simulink model "Dyn_6DoF_v2_0_R2015B"  (R2015b)
settings: Solver=ode4  SolverMode=SingleTasking  StartTime=0.0  StopTime=simInit.TSIM  FixedStep=simInit.dt  MaxStep=simInit.dt  RelTol=1e-3
InitFcn:
  | close all
undefined symbols (not defined in the file): act, base_windspeed, constr, DE2019, DiscIntNeverNeededParam, ENVMT, Lbooth, loiterStates, omega_rate_max, params, simInit, T, winchParameter
libraries: simulink x41, simulink_extras x4, dspsigops x1
(part 1 of 6)
Description:
  | % Copyright 2020 Delft University of Technology
  | %
  | % Licensed under the Apache License, Version 2.0 (the "License");
  | % you may not use this file except in compliance with the License.
  | % You may obtain a copy of the License at
  | %
  | %      http://www.apache.org/licenses/LICENSE-2.0
  | %
  | % Unless required by applicable law or agreed to in writing, software
  | % distributed under the License is distributed on an "AS IS" BASIS,
  | % WITHOUT WARRANTIES OR CONDITIONS OF ANY KIND, either express or implied.
  | % See the License for the specific language governing permissions and
  | % limitations under the License.
settings Model: SimulationMode=accelerator  NumberOfSteps=50  ExtModeTrigDuration=100  Creator=Sebastian  LastModifiedBy=dylaneijkelhof
settings SolverCC: SolverJacobianMethodControl=FullAnalytical
settings DataIOCC: InitialState=testPoint  LimitDataPoints=off  SaveFormat=Structure  SignalLogging=off  DSMLogging=off  SaveTime=off  StateSaveName=tmp_raccel_xout  SignalLoggingName=logged_signals
settings OptimizationCC: BlockReduction=off  EfficientMapNaN2IntZero=off
settings DebuggingCC: ArtificialAlgebraicLoopMsg=none  SaveWithDisabledLinksMsg=none  SaveWithParameterizedLinksMsg=none  MaskedZcDiagnostic=none  IgnoredZcDiagnostic=none  InheritedTsInSrcMsg=none  TasksWithSamePriorityMsg=none  SigSpecEnsureSampleTimeMsg=none  ParameterPrecisionLossMsg=none  UnconnectedInputMsg=none  UnconnectedOutputMsg=none  UnconnectedLineMsg=none  BusObjectLabelMismatch=none  RootOutportRequireBusObject=none  AllowSymbolicDim=on  UnknownTsInhSupMsg=none  ModelReferenceDataLoggingMessage=none  ModelReferenceSymbolNameMessage=none  InitInArrayFormatMsg=none  SFUnusedDataAndEventsDiag=none  SFUnexpectedBacktrackingDiag=none  SFInvalidInputDataAccessInChartInitDiag=none  SFNoUnconditionalDefaultTransitionDiag=none  SFTransitionOutsideNaturalParentDiag=none  SFUnconditionalTransitionShadowingDiag=none  SFUndirectedBroadcastEventsDiag=none  SFTransitionActionBeforeConditionDiag=none
settings HardwareCC: ProdBitPerLong=64  ProdLongLongMode=on  ProdHWDeviceType=Custom Processor->Custom Processor  TargetBitPerLong=64  TargetBitPerPointer=64  TargetLargestAtomicFloat=Float  TargetLongLongMode=on  TargetIntDivRoundTo=Zero  TargetEndianess=LittleEndian  TargetWordSize=64  TargetHWDeviceType=Custom Processor->MATLAB Host Computer
settings RTWCC: RTWUseLocalCustomCode=on
settings CodeAppCC: MaxIdLength=128
settings GRTTargetCC: CombineOutputUpdateFcns=off  GRTInterface=on
settings ConfigComp: CovModelRefEnable=Off
settings SimscapeCC: SimscapeNormalizeSystem=off

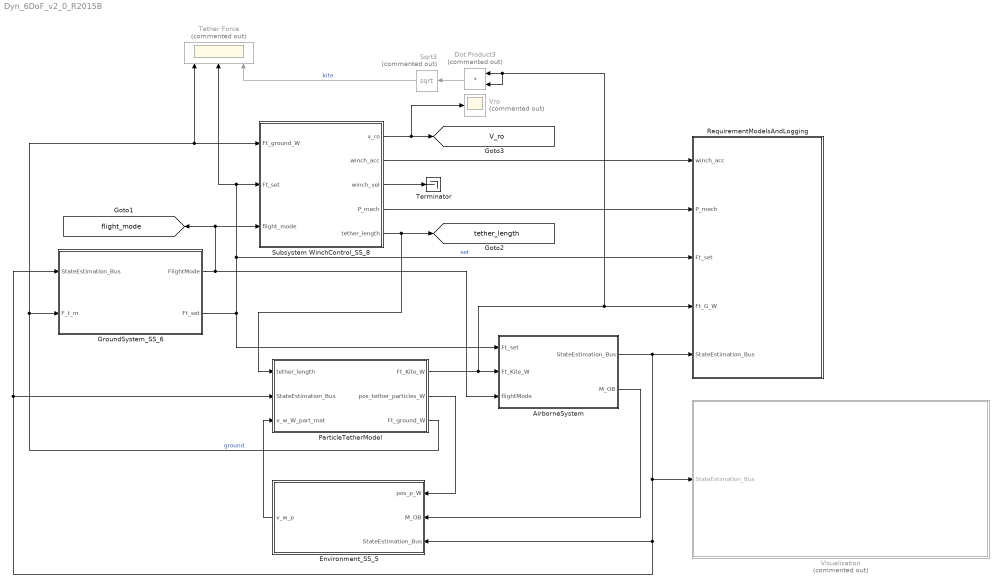
== system Dyn_6DoF_v2_0_R2015B ==
  AirborneSystem : Subsystem
  Dot Product3 : DotProduct  Commented=on  InputSameDT=on  OutDataTypeStr=Inherit: Inherit via internal rule
  Environment_SS_5 : Subsystem
  GroundSystem_SS_6 : Subsystem
  ParticleTetherModel : Subsystem
  RequirementModelsAndLogging : Subsystem  mask{log_sample_time=0.2}
  Sqrt3 : Sqrt  Commented=on  SaturateOnIntegerOverflow=on
  Subsystem WinchControl_SS_8 : Subsystem
  Terminator : Terminator
  Tether Force : Scope  Commented=on  NumInputPorts=3
  Visualisation : Subsystem  Commented=on  mask{sample_time_vis=1}
      mask prompts: sample_time_vis "sampletime"
      mask Display: image('DE2019_Aircraft.jpeg')
  Vro : Scope  Commented=on
  tag scope: V_ro=global, flight_mode=global, tether_length=global
  wires:
  GroundSystem_SS_6/1(FlightMode) -> AirborneSystem/3(flightMode), Subsystem WinchControl_SS_8/3(flight_mode), [flight_mode]
  GroundSystem_SS_6/2(Ft_set) -> Subsystem WinchControl_SS_8/2(Ft_set), Tether Force/2, RequirementModelsAndLogging/3(Ft_set), AirborneSystem/1(Ft_set)  "set"
  AirborneSystem/2(M_OB) -> Environment_SS_5/2(M_OB)
  AirborneSystem/1(StateEstimation_Bus) -> RequirementModelsAndLogging/5(StateEstimation_Bus), Environment_SS_5/3(StateEstimation_Bus), GroundSystem_SS_6/1(StateEstimation_Bus), ParticleTetherModel/2(StateEstimation_Bus), Visualisation/1(StateEstimation_Bus)
  ParticleTetherModel/2(pos_tether_particles_W) -> Environment_SS_5/1(pos_p_W)
  Environment_SS_5/1(v_w_p) -> ParticleTetherModel/3(v_w_W_part_mat)
  Subsystem WinchControl_SS_8/1(v_ro) -> Vro/1, [V_ro]
  ParticleTetherModel/3(Ft_ground_W) -> GroundSystem_SS_6/2(F_t_m), Subsystem WinchControl_SS_8/1(Ft_ground_W), Tether Force/1  "ground"
  Subsystem WinchControl_SS_8/3(winch_vel) -> Terminator/1
  Subsystem WinchControl_SS_8/2(winch_acc) -> RequirementModelsAndLogging/1(winch_acc)
  Subsystem WinchControl_SS_8/4(P_mech) -> RequirementModelsAndLogging/2(P_mech)
  Subsystem WinchControl_SS_8/5(tether_length) -> [tether_length], ParticleTetherModel/1(tether_length)
  Sqrt3/1 -> Tether Force/3  "kite"
  Dot Product3/1 -> Sqrt3/1
  ParticleTetherModel/1(Ft_Kite_W) -> RequirementModelsAndLogging/4(Ft_G_W), Dot Product3/2, Dot Product3/1, AirborneSystem/2(Ft_Kite_W)

== system Dyn_6DoF_v2_0_R2015B/AirborneSystem ==
  Ft_set : Inport
  Ft_Kite_W : Inport  Port=2
  flightMode : Inport  Port=3
  6DoFDynamics : Subsystem
  Dot Product : DotProduct  InputSameDT=on  OutDataTypeStr=Inherit: Inherit via internal rule
  FlightControlSystem : Subsystem
  ForcesAndTorques : Subsystem
  Sqrt : Sqrt  SaturateOnIntegerOverflow=on
  StateEstimation_Bus : Outport
  M_OB : Outport  Port=2
  wires:
  6DoFDynamics/2(StateEstimation_Bus) -> FlightControlSystem/4(StateEstimation_Bus), ForcesAndTorques/3(StateEstimation_Bus), StateEstimation_Bus/1  "StateEstimation_Bus"
  6DoFDynamics/1(M_OB) -> M_OB/1
  Ft_Kite_W/1 -> 6DoFDynamics/1(F_t_W), Dot Product/2, Dot Product/1
  Dot Product/1 -> Sqrt/1
  Ft_set/1 -> FlightControlSystem/2(Ft_set)
  Sqrt/1 -> FlightControlSystem/3(Ft_tot_kite)
  ForcesAndTorques/1(F_a_B) -> 6DoFDynamics/2(F_a_B), FlightControlSystem/1(F_a_B)
  FlightControlSystem/2(throttle/brake) -> ForcesAndTorques/2(throttle/brake)
  ForcesAndTorques/2(F_p_B) -> 6DoFDynamics/3(F_p_B)
  ForcesAndTorques/3(M_a_B) -> 6DoFDynamics/4(Torques), FlightControlSystem/5(M_a_B)
  FlightControlSystem/1(u_controlsurfaces) -> ForcesAndTorques/1(u_cmd)
  flightMode/1 -> FlightControlSystem/6(fm)

== system Dyn_6DoF_v2_0_R2015B/Environment_SS_5 ==
  note: Tether
  note: Kite
  note: note: wind field calc occurs twice, here and in windshear
  pos_p_W : Inport
  M_OB : Inport  Port=2
  StateEstimation_Bus : Inport  Port=3
  Bus Selector : BusSelector  OutputSignals=pos_G_O_m
  Constant4 : Constant  Value=ENVMT.windDirection_rad
  Delay : Delay  DelayLength=1  InitialCondition=zeros(3,1)
  Gain : Gain  Gain=-1
  Gain1 : Gain  Gain=-1
  MATLAB Function : MATLAB Function  TreatAsAtomicUnit=on
  MATLAB Function1 : MATLAB Function  TreatAsAtomicUnit=on
  Product : Product  Multiplication=Matrix(*)
  Reshape1 : Reshape  OutputDimensionality=Column vector (2-D)
  Selector : Selector  InputPortWidth=3  IndexOptions=Index vector (dialog)  Indices=3  OutputSizes=1
  Wdeg2 : Constant  Value=base_windspeed  OutDataTypeStr=Inherit: Inherit via back propagation
  Windshear : Subsystem
  wind_field_calc : Subsystem
  v_w_p : Outport
  tag scope: vel_W_W=global
  wires:
  wind_field_calc/1(Windspeed_altitude) -> MATLAB Function1/1(v_w_u)
  Wdeg2/1 -> wind_field_calc/2(Base_windspeed)
  Delay/1 -> [vel_W_W]
  MATLAB Function1/1(v_w_p_mat) -> v_w_p/1
  pos_p_W/1 -> wind_field_calc/1(Altitude)
  Reshape1/1 -> Delay/1
  Constant4/1 -> MATLAB Function/2(wind_direction_rad)
  Gain/1 -> Windshear/2(altitude)
  Gain1/1 -> Product/2
  Windshear/1(V_shear_mDs) -> Gain1/1
  M_OB/1 -> Windshear/1(DCM), Product/1
  Product/1 -> MATLAB Function/1(vec_O)
  StateEstimation_Bus/1 -> Bus Selector/1
  MATLAB Function/1(vec_W) -> Reshape1/1
  Selector/1 -> Gain/1
  Bus Selector/1 -> Selector/1  "<pos_G_O_m>"

== system Dyn_6DoF_v2_0_R2015B/GroundSystem_SS_6 ==
  StateEstimation_Bus : Inport
  F_t_m : Inport  Port=2
  Bus Selector : BusSelector  OutputSignals=pos_G_W,airdata,longlat,pathangles_k
  Demux : Demux  Outputs=2
  Demux1 : Demux  Outputs=2
  GroundControl : Subsystem
  Selector : Selector  InputPortWidth=3  IndexOptions=Index vector (dialog)  Indices=1  OutputSizes=1
  Selector1 : Selector  InputPortWidth=3  IndexOptions=Index vector (dialog)  Indices=1  OutputSizes=1
  Selector3 : Selector  InputPortWidth=2  IndexOptions=Index vector (dialog)  Indices=1  OutputSizes=1
  StateMachine : Subsystem
  Terminator : Terminator
  FlightMode : Outport
  Ft_set : Outport  Port=2
  tag scope: phi0_update=global
  wires:
  Demux1/1 -> StateMachine/9(Chi)
  Demux1/2 -> Terminator/1
  Bus Selector/4 -> Demux1/1  "<pathangles_k>"
  GroundControl/2(lat_init) -> StateMachine/8(lat_init)
  Selector3/1 -> GroundControl/2(long)
  GroundControl/1(path_update) -> Selector1/1, StateMachine/5(path_update)
  Selector1/1 -> [phi0_update]
  StateMachine/1(FlightMode) -> FlightMode/1, GroundControl/1(flightMode)
  Bus Selector/3 -> Selector3/1, Demux/1  "<longlat>"
  F_t_m/1 -> StateMachine/7(F_t_m)
  [cross_track_error] -> StateMachine/6(cross_track_error)
  Demux/2 -> StateMachine/4(lattitude)
  StateMachine/2(Ft_set) -> Ft_set/1
  Demux/1 -> StateMachine/3(longitude)
  StateEstimation_Bus/1 -> Bus Selector/1
  Bus Selector/1 -> StateMachine/1(pos_W)  "<pos_G_W>"
  Bus Selector/2 -> Selector/1  "<airdata>"
  Selector/1 -> StateMachine/2(Va)

== system Dyn_6DoF_v2_0_R2015B/ParticleTetherModel ==
  tether_length : Inport
  StateEstimation_Bus : Inport  Port=2
  v_w_W_part_mat : Inport  Port=3
  Bus Selector : BusSelector  OutputSignals=pos_G_W,vel_W
  Dot Product2 : DotProduct  Commented=on  InputSameDT=on  OutDataTypeStr=Inherit: Inherit via internal rule
  Selector : Selector  NumberOfDimensions=2  InputPortWidth=3  IndexOptions=Index vector (dialog),Select all  Indices=1,1  OutputSizes=1,1
  Selector4 : Selector  NumberOfDimensions=2  InputPortWidth=3  IndexOptions=Index vector (dialog),Select all  Indices=2,1  OutputSizes=1,1
  Selector5 : Selector  NumberOfDimensions=2  InputPortWidth=3  IndexOptions=Index vector (dialog),Select all  Indices=3,1  OutputSizes=1,1
  Sqrt2 : Sqrt  Commented=on  SaturateOnIntegerOverflow=on
  Tether_SS_7 : Subsystem
  Transpose : Math  Operator=transpose  SaturateOnIntegerOverflow=on
  Transpose1 : Math  Operator=transpose  SaturateOnIntegerOverflow=on
  Transpose2 : Math  Operator=transpose  SaturateOnIntegerOverflow=on
  error tether : Scope  Commented=on
  Ft_Kite_W : Outport
  pos_tether_particles_W : Outport  Port=2
  Ft_ground_W : Outport  Port=3
  tag scope: p_t_x=global, p_t_y=global, p_t_z=global
  wires:
  v_w_W_part_mat/1 -> Tether_SS_7/3(windVel)
  StateEstimation_Bus/1 -> Bus Selector/1
  Bus Selector/1 -> Tether_SS_7/1(pos_G_W)  "<pos_G_W>"
  Bus Selector/2 -> Tether_SS_7/2(vel_W)  "<vel_W>"
  Selector4/1 -> Transpose1/1
  Selector5/1 -> Transpose2/1
  Selector/1 -> Transpose/1
  Transpose/1 -> [p_t_x]
  Transpose1/1 -> [p_t_y]
  Transpose2/1 -> pos_tether_particles_W/1, [p_t_z]
  Tether_SS_7/4(Error_3D) -> Dot Product2/2, Dot Product2/1
  Tether_SS_7/1(x tether W) -> Selector/1, Selector5/1, Selector4/1
  Dot Product2/1 -> Sqrt2/1
  Sqrt2/1 -> error tether/1
  Tether_SS_7/2(Ft_Ground) -> Ft_ground_W/1
  Tether_SS_7/3(Ft_Kite) -> Ft_Kite_W/1
  tether_length/1 -> Tether_SS_7/4(tetherLength)

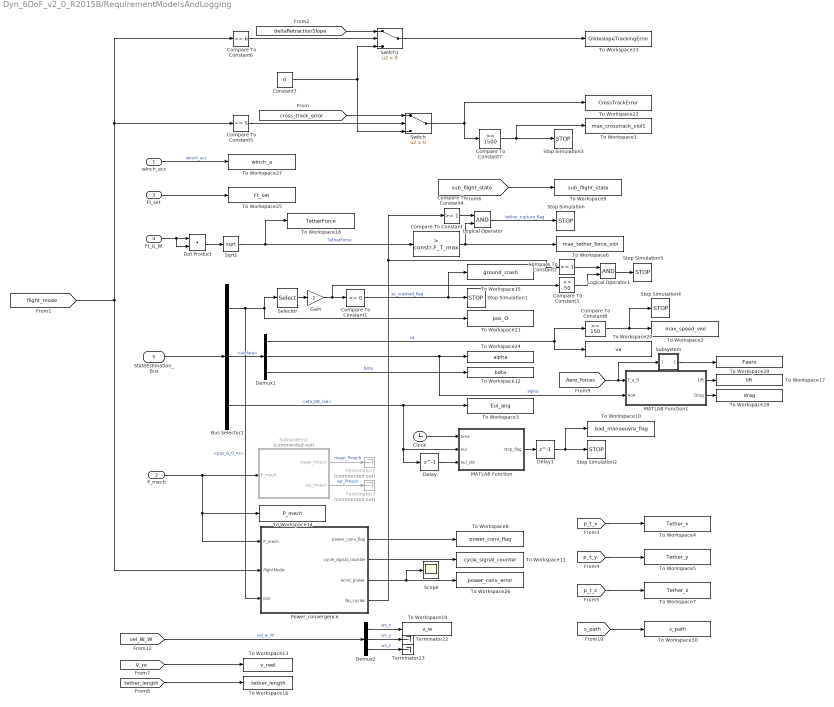
== system Dyn_6DoF_v2_0_R2015B/RequirementModelsAndLogging ==
  winch_acc : Inport
  P_mech : Inport  Port=2
  Ft_set : Inport  Port=3
  Ft_G_W : Inport  Port=4
  StateEstimation_Bus : Inport  Port=5
  Bus Selector1 : BusSelector  OutputSignals=pos_G_O_m,airdata,eta_OB_rad
  Clock : Clock
  Compare To Constant : simulink/Logic and Bit Operations/Compare To Constant  relop=>  const=constr.F_T_max  OutDataTypeStr=boolean
  Compare To Constant1 : simulink/Logic and Bit Operations/Compare To Constant  relop=<=  const=0  OutDataTypeStr=boolean
  Compare To Constant2 : simulink/Logic and Bit Operations/Compare To Constant  relop=>=  const=1  OutDataTypeStr=boolean
  Compare To Constant3 : simulink/Logic and Bit Operations/Compare To Constant  relop=<=  const=50  OutDataTypeStr=boolean
  Compare To Constant4 : simulink/Logic and Bit Operations/Compare To Constant  relop=>=  const=1  OutDataTypeStr=boolean
  Compare To Constant5 : simulink/Logic and Bit Operations/Compare To Constant  relop===  const=5  OutDataTypeStr=boolean
  Compare To Constant6 : simulink/Logic and Bit Operations/Compare To Constant  relop===  const=6  OutDataTypeStr=boolean
  Compare To Constant7 : simulink/Logic and Bit Operations/Compare To Constant  relop=>=  const=1500  OutDataTypeStr=boolean
  Compare To Constant8 : simulink/Logic and Bit Operations/Compare To Constant  relop=>=  const=150  OutDataTypeStr=boolean
  Constant7 : Constant  Value=0
  Delay : Delay  DelayLength=1  InitialCondition=zeros(3,1)
  Delay1 : Delay  DelayLength=1
  Demux1 : Demux  Outputs=3
  Demux2 : Demux  Outputs=3
  Dot Product : DotProduct  InputSameDT=on  OutDataTypeStr=Inherit: Inherit via internal rule
  Gain : Gain  Gain=-1
  Logical Operator : Logic  AllPortsSameDT=off  OutDataTypeStr=boolean
  Logical Operator1 : Logic  AllPortsSameDT=off  OutDataTypeStr=boolean
  MATLAB Function : MATLAB Function  TreatAsAtomicUnit=on
  MATLAB Function1 : MATLAB Function  TreatAsAtomicUnit=on
  Power_convergence : Subsystem  mask{sample_time=simInit.Ts_power_conv_check, threshold=130000, min_cycles=3, pos_threshold=400}
      mask prompts: threshold "start_threshold"; min_cycles "minimum_cycles"; pos_threshold "maximum position distance"
  Scope : Scope
  Selector : Selector  InputPortWidth=3  IndexOptions=Index vector (dialog)  Indices=3  OutputSizes=1
  Sqrt1 : Sqrt  SaturateOnIntegerOverflow=on
  Stop Simulation{,1..5} (6 alike) : Stop
  Subsystem : Subsystem
      mask Display: disp('norm()')
  Subsystem2 : Subsystem  Commented=on
  Switch : Switch  Criteria=u2 > Threshold
  Switch1 : Switch  Criteria=u2 > Threshold
  Terminator1 : Terminator  Commented=on
  Terminator22 : Terminator
  Terminator23 : Terminator
  Terminator7 : Terminator  Commented=on
  To Workspace1 : ToWorkspace  VariableName=max_crosstrack_viol1  SampleTime=-1
      settings: MaxDataPoints=1
  To Workspace10 : ToWorkspace  VariableName=bad_manoeuvre_flag  SampleTime=-1
      settings: MaxDataPoints=1
  To Workspace11 : ToWorkspace  VariableName=cycle_signal_counter  SaveFormat=Timeseries  SampleTime=-1
      settings: MaxDataPoints=1  Save2DSignal=2-D array (concatenate along first dimension)
  To Workspace12 : ToWorkspace  VariableName=beta  SaveFormat=Timeseries  SampleTime=simInit.AttLoggingTs
      settings: Save2DSignal=2-D array (concatenate along first dimension)
  To Workspace13 : ToWorkspace  VariableName=v_reel  SaveFormat=Timeseries  SampleTime=simInit.PLoggingTs
  To Workspace14 : ToWorkspace  VariableName=P_mech  SaveFormat=Timeseries  SampleTime=simInit.PLoggingTs
  To Workspace15 : ToWorkspace  VariableName=ground_crash  SampleTime=-1
      settings: MaxDataPoints=1
  To Workspace16 : ToWorkspace  VariableName=tether_length  SaveFormat=Timeseries  SampleTime=simInit.AttLoggingTs
  To Workspace17 : ToWorkspace  VariableName=lift  SaveFormat=Timeseries  SampleTime=simInit.AttLoggingTs
      settings: Save2DSignal=2-D array (concatenate along first dimension)
  To Workspace18 : ToWorkspace  VariableName=TetherForce  SaveFormat=Timeseries  SampleTime=simInit.FtLoggingTs
  To Workspace19 : ToWorkspace  VariableName=v_w  SaveFormat=Timeseries  SampleTime=simInit.PLoggingTs
  To Workspace2 : ToWorkspace  VariableName=max_speed_viol  SampleTime=-1
      settings: MaxDataPoints=1
  To Workspace20 : ToWorkspace  VariableName=va  SaveFormat=Timeseries  SampleTime=simInit.AttLoggingTs
      settings: Save2DSignal=2-D array (concatenate along first dimension)
  To Workspace21 : ToWorkspace  VariableName=pos_O  SaveFormat=Timeseries  SampleTime=simInit.PLoggingTs
      settings: Save2DSignal=2-D array (concatenate along first dimension)
  To Workspace22 : ToWorkspace  VariableName=CrossTrackError  SaveFormat=Timeseries  SampleTime=simInit.CteLoggingTs
      settings: Save2DSignal=2-D array (concatenate along first dimension)
  To Workspace23 : ToWorkspace  VariableName=GlideslopeTrackingError  SaveFormat=Timeseries  SampleTime=simInit.GSLoggingTs
      settings: Save2DSignal=2-D array (concatenate along first dimension)
  To Workspace24 : ToWorkspace  VariableName=alpha  SaveFormat=Timeseries  SampleTime=simInit.AttLoggingTs
      settings: Save2DSignal=2-D array (concatenate along first dimension)
  To Workspace25 : ToWorkspace  VariableName=Ft_set  SaveFormat=Timeseries  SampleTime=simInit.FtLoggingTs
  To Workspace26 : ToWorkspace  VariableName=power_conv_error  SaveFormat=Timeseries  SampleTime=-1
      settings: Save2DSignal=2-D array (concatenate along first dimension)
  To Workspace27 : ToWorkspace  VariableName=winch_a  SaveFormat=Timeseries  SampleTime=simInit.PLoggingTs
  To Workspace28 : ToWorkspace  VariableName=drag  SaveFormat=Timeseries  SampleTime=simInit.AttLoggingTs
      settings: Save2DSignal=2-D array (concatenate along first dimension)
  To Workspace29 : ToWorkspace  VariableName=Faero  SaveFormat=Timeseries  SampleTime=simInit.AttLoggingTs
      settings: Save2DSignal=2-D array (concatenate along first dimension)
  To Workspace3 : ToWorkspace  VariableName=Eul_ang  SaveFormat=Timeseries  SampleTime=simInit.PLoggingTs
      settings: Save2DSignal=2-D array (concatenate along first dimension)
  To Workspace30 : ToWorkspace  VariableName=s_path  SaveFormat=Timeseries  SampleTime=simInit.PLoggingTs
      settings: Save2DSignal=2-D array (concatenate along first dimension)
  To Workspace4 : ToWorkspace  VariableName=Tether_x  SaveFormat=Timeseries  SampleTime=simInit.PLoggingTs
      settings: Save2DSignal=2-D array (concatenate along first dimension)
  To Workspace5 : ToWorkspace  VariableName=Tether_y  SaveFormat=Timeseries  SampleTime=simInit.PLoggingTs
      settings: Save2DSignal=2-D array (concatenate along first dimension)
  To Workspace6 : ToWorkspace  VariableName=max_tether_force_viol  SampleTime=-1
      settings: MaxDataPoints=1
  To Workspace7 : ToWorkspace  VariableName=Tether_z  SaveFormat=Timeseries  SampleTime=simInit.PLoggingTs
      settings: Save2DSignal=2-D array (concatenate along first dimension)
  To Workspace8 : ToWorkspace  VariableName=power_conv_flag  SampleTime=-1
      settings: MaxDataPoints=1
  To Workspace9 : ToWorkspace  VariableName=sub_flight_state  SaveFormat=Timeseries  SampleTime=simInit.FtLoggingTs
  wires:
  Bus Selector1/1 -> Power_convergence/3(pos), Selector/1, To Workspace21/1  "<pos_G_O_m>"
  Gain/1 -> Compare To Constant3/1, Compare To Constant1/1
  Compare To Constant1/1 -> To Workspace15/1, Stop Simulation1/1  "ac_crashed_flag"
  Selector/1 -> Gain/1
  winch_acc/1 -> To Workspace27/1  "winch_acc"
  Logical Operator/1 -> Stop Simulation/1  "tether_rupture_flag"
  Sqrt1/1 -> To Workspace18/1, Compare To Constant/1  "TetherForce"
  StateEstimation_Bus/1 -> Bus Selector1/1
  Power_convergence/1(power_conv_flag) -> To Workspace8/1
  Power_convergence/2(cycle_signal_counter) -> To Workspace11/1
  [vel_W_W] -> Demux2/1  "vel_w_W"
  Bus Selector1/2 -> Demux1/1  "<airdata>"
  Switch/1 -> To Workspace22/1, Compare To Constant7/1
  Subsystem2/1(mean_Pmech) -> Terminator1/1  "mean_Pmech"
  Subsystem2/2(var_Pmech) -> Terminator7/1  "var_Pmech"
  Demux1/1 -> To Workspace20/1, Compare To Constant8/1  "va"
  Demux1/2 -> MATLAB Function1/2(AoA), To Workspace24/1  "alpha"
  Demux1/3 -> To Workspace12/1  "beta"
  Demux2/3 -> Terminator23/1  "ws_z"
  Demux2/2 -> Terminator22/1  "ws_y"
  Demux2/1 -> To Workspace19/1  "ws_x"
  Ft_G_W/1 -> Dot Product/2, Dot Product/1
  Dot Product/1 -> Sqrt1/1
  Clock/1 -> MATLAB Function/1(time)
  Compare To Constant4/1 -> Logical Operator/1
  Compare To Constant/1 -> Logical Operator/2, To Workspace6/1
  [flight_mode] -> Compare To Constant6/1, Compare To Constant5/1, Power_convergence/2(flightMode)
  P_mech/1 -> Power_convergence/1(P_mech), To Workspace14/1, Subsystem2/1(P_mech)
  Compare To Constant5/1 -> Switch/2
  [cross_track_error] -> Switch/1
  Switch1/1 -> To Workspace23/1
  [deltaRetractionSlope] -> Switch1/1
  Compare To Constant6/1 -> Switch1/2
  Constant7/1 -> Switch1/3, Switch/3
  Ft_set/1 -> To Workspace25/1
  Power_convergence/3(error_power) -> Scope/1, To Workspace26/1
  Compare To Constant7/1 -> Stop Simulation3/1, To Workspace1/1
  Compare To Constant8/1 -> To Workspace2/1, Stop Simulation4/1
  Bus Selector1/3 -> Delay/1, MATLAB Function/2(eul), To Workspace3/1  "<eta_OB_rad>"
  [p_t_y] -> To Workspace5/1
  [p_t_x] -> To Workspace4/1
  [p_t_z] -> To Workspace7/1
  [sub_flight_state] -> To Workspace9/1
  Delay/1 -> MATLAB Function/3(eul_old)
  MATLAB Function/1(stop_flag) -> Delay1/1
  Delay1/1 -> Stop Simulation2/1, To Workspace10/1
  [V_ro] -> To Workspace13/1
  [tether_length] -> To Workspace16/1
  [Aero_forces] -> Subsystem/1(In1), MATLAB Function1/1(F_a_B)
  MATLAB Function1/1(Lift) -> To Workspace17/1
  MATLAB Function1/2(Drag) -> To Workspace28/1
  Power_convergence/4(No_cycles) -> Compare To Constant2/1, Compare To Constant4/1
  Compare To Constant2/1 -> Logical Operator1/1
  Compare To Constant3/1 -> Logical Operator1/2
  Logical Operator1/1 -> Stop Simulation5/1
  Subsystem/1(Out1) -> To Workspace29/1
  [s_path] -> To Workspace30/1

== system Dyn_6DoF_v2_0_R2015B/Subsystem WinchControl_SS_8 ==
  Ft_ground_W : Inport  OutDataTypeStr=double  PortDimensions=1
  Ft_set : Inport  Port=2  OutDataTypeStr=double  PortDimensions=1
  flight_mode : Inport  Port=3  OutDataTypeStr=double  PortDimensions=1
  Compare To Constant1 : simulink/Logic and Bit Operations/Compare To Constant  relop===  const=6  OutDataTypeStr=boolean
  Gain1 : Gain  Gain=winchParameter.radius
  Power : Scope
  Product : Product
  PureTorqueControl : Subsystem
  Reel-out speed : Scope
  Scope : Scope  Commented=on
  Winch acc : Scope
  WinchDynamics : Subsystem
  tether length : Scope
  v_ro : Outport  OutDataTypeStr=double  PortDimensions=1
  winch_acc : Outport  Port=2  OutDataTypeStr=double  PortDimensions=1
  winch_vel : Outport  Port=3  OutDataTypeStr=double  PortDimensions=1
  P_mech : Outport  Port=4  OutDataTypeStr=double  PortDimensions=1
  tether_length : Outport  Port=5  OutDataTypeStr=double  PortDimensions=1
  wires:
  Gain1/1 -> Product/2, Reel-out speed/1, v_ro/1
  WinchDynamics/2(theta_dot) -> PureTorqueControl/4(theta_dot), Gain1/1
  Ft_ground_W/1 -> PureTorqueControl/1(F_t_m_grnd), Product/1, WinchDynamics/1(for_tether_tot)
  WinchDynamics/4(winch_vel) -> winch_vel/1
  Product/1 -> Power/1, P_mech/1  "P_mech"
  Ft_set/1 -> PureTorqueControl/3(F_t_set)
  flight_mode/1 -> Compare To Constant1/1
  WinchDynamics/3(winch_acc) -> Winch acc/1, winch_acc/1
  WinchDynamics/1(tether_length) -> tether_length/1, tether length/1
  PureTorqueControl/1(torque_cmd) -> Scope/1, WinchDynamics/2(control_moments)
  Compare To Constant1/1 -> PureTorqueControl/2(retraction_flag)

== system Dyn_6DoF_v2_0_R2015B/Visualisation ==
  StateEstimation_Bus : Inport
  Bus Selector1 : BusSelector  OutputSignals=pos_G_O_m,eta_OB_rad
  Clock : Clock
  Constant5 : Constant  Value=sample_time_vis
  Visualisation : MATLAB Function  TreatAsAtomicUnit=on
  wires:
  Clock/1 -> Visualisation/1(t)
  Bus Selector1/2 -> Visualisation/7(eta_OB)  "<eta_OB_rad>"
  [phi0_update] -> Visualisation/5(phi0_update)
  Bus Selector1/1 -> Visualisation/6(pos_O)  "<pos_G_O_m>"
  [p_t_y] -> Visualisation/3(p_t_y)
  StateEstimation_Bus/1 -> Bus Selector1/1
  [p_t_z] -> Visualisation/4(p_t_z)
  [p_t_x] -> Visualisation/2(p_t_x)
  [sub_flight_state] -> Visualisation/8(sub_flight_state)
  Constant5/1 -> Visualisation/10(sampletime)
  [arcP] -> Visualisation/9(arcP)

== system Dyn_6DoF_v2_0_R2015B/AirborneSystem/6DoFDynamics ==
  F_t_W : Inport
  F_a_B : Inport  Port=2
  F_p_B : Inport  Port=3
  Torques : Inport  Port=4
  Bus Creator1 : BusCreator  Inputs=15
  Delay1 : Delay  DelayLength=1
  Demux : Demux  Outputs=3
  Dot Product : DotProduct  Commented=on  InputSameDT=on  OutDataTypeStr=Inherit: Inherit via internal rule
  Dot Product1 : DotProduct  InputSameDT=on  OutDataTypeStr=Inherit: Inherit via internal rule
  MATLAB Function3 : MATLAB Function  TreatAsAtomicUnit=on
  Mux1 : Mux  Inputs=3
  Sqrt : Sqrt  Commented=on  SaturateOnIntegerOverflow=on
  Sqrt1 : Sqrt  SaturateOnIntegerOverflow=on
  Subsystem : Subsystem
  Vk : Scope  Commented=on
  M_OB : Outport  PortDimensions=[3,3]
  StateEstimation_Bus : Outport  Port=2
  wires:
  Demux/1 -> Bus Creator1/9  "mu_a"
  Subsystem/15(M_OB) -> M_OB/1
  Subsystem/8(Va) -> Mux1/1
  Subsystem/1(pathangles_a) -> Bus Creator1/1  "pathangles_a"
  [vel_W_W] -> Subsystem/4(v_w_W)
  Torques/1 -> Subsystem/3(Torques_B)
  F_p_B/1 -> Subsystem/2(F_p_B)
  F_a_B/1 -> Subsystem/1(F_a_B)
  Subsystem/4(pathangles_k) -> Bus Creator1/4  "pathangles_k"
  Subsystem/2(v_k_B) -> Bus Creator1/2, Dot Product/1, Dot Product/2  "v_k_B"
  Subsystem/10(EULER) -> Bus Creator1/10  "eta_OB_rad"
  Subsystem/6(longlat) -> Bus Creator1/6  "longlat"
  Subsystem/5(vel_K_O_mDs) -> Bus Creator1/5  "vel_K_O_mDs"
  Bus Creator1/1 -> StateEstimation_Bus/1
  Subsystem/3(omega_OB_B) -> Bus Creator1/3  "omega_OB_B"
  Subsystem/7(pos_O) -> Bus Creator1/7  "pos_G_O_m"
  Demux/3 -> Mux1/3
  Subsystem/9(eta_a) -> Demux/1
  Delay1/1 -> Bus Creator1/12  "a_tot"
  Sqrt1/1 -> Delay1/1
  Dot Product1/1 -> Sqrt1/1
  Subsystem/12(a_B) -> Dot Product1/1, Dot Product1/2
  Subsystem/11(mu_k) -> Bus Creator1/11  "mu_k"
  MATLAB Function3/1(v_w_O) -> Bus Creator1/15  "v_w_hat_O"
  [vel_W_W] -> MATLAB Function3/1(v_w_W)
  Mux1/1 -> Bus Creator1/8  "airdata"
  Demux/2 -> Mux1/2
  F_t_W/1 -> Subsystem/5(F_t_W)
  Subsystem/13(pos_W) -> Bus Creator1/13  "pos_G_W"
  Subsystem/14(vel_W) -> Bus Creator1/14  "vel_W"
  Sqrt/1 -> Vk/1
  Dot Product/1 -> Sqrt/1

== system Dyn_6DoF_v2_0_R2015B/AirborneSystem/FlightControlSystem ==
  F_a_B : Inport
  Ft_set : Inport  Port=2
  Ft_tot_kite : Inport  Port=3
  StateEstimation_Bus : Inport  Port=4
  M_a_B : Inport  Port=5
  fm : Inport  Port=6
  AirspeedController_SS_1 : Subsystem
  AoA : Scope  NumInputPorts=2
  AttitudeAndRateLoop : Subsystem
  Bus Selector : BusSelector  OutputSignals=airdata,pathangles_a,v_k_B
  PathFollowingController_SS_3 : Subsystem
  Selector : Selector  InputPortWidth=3  IndexOptions=Index vector (dialog)  Indices=1  OutputSizes=1
  Selector1 : Selector  InputPortWidth=3  IndexOptions=Index vector (dialog)  Indices=2  OutputSizes=1
  Selector2 : Selector  InputPortWidth=2  IndexOptions=Index vector (dialog)  Indices=2  OutputSizes=1
  Va : Scope
  u_controlsurfaces : Outport
  throttle/brake : Outport  Port=2
  wires:
  StateEstimation_Bus/1 -> PathFollowingController_SS_3/4(StateEstimation_Bus), Bus Selector/1, AttitudeAndRateLoop/5(StateEstimation_Bus)
  Ft_set/1 -> PathFollowingController_SS_3/1(ft_set)
  Ft_tot_kite/1 -> AirspeedController_SS_1/6(Ft_set), PathFollowingController_SS_3/2(f_t_kite)
  Bus Selector/1 -> Selector/1, Selector1/1  "<airdata>"
  Selector2/1 -> AirspeedController_SS_1/3(gamma_a)
  Selector/1 -> AirspeedController_SS_1/1(Va), Va/1
  Selector1/1 -> AirspeedController_SS_1/2(alpha), AoA/1
  F_a_B/1 -> AirspeedController_SS_1/5(F_a_B), PathFollowingController_SS_3/3(F_a_B_est)
  Bus Selector/2 -> Selector2/1  "<pathangles_a>"
  AirspeedController_SS_1/1(Thrust_Brake_force) -> throttle/brake/1
  AttitudeAndRateLoop/1(u_rb) -> u_controlsurfaces/1
  PathFollowingController_SS_3/1(mu_a_cmd) -> AttitudeAndRateLoop/1(mu_a_cmd)
  PathFollowingController_SS_3/2(alpha_a_cmd) -> AttitudeAndRateLoop/4(alpha_a_cmd), AoA/2
  M_a_B/1 -> AttitudeAndRateLoop/2(M_a_B_est)
  fm/1 -> AttitudeAndRateLoop/3(flightMode)
  Bus Selector/3 -> AirspeedController_SS_1/4(V_k_B)  "<v_k_B>"

== system Dyn_6DoF_v2_0_R2015B/AirborneSystem/ForcesAndTorques ==
  u_cmd : Inport
  throttle/brake : Inport  Port=2
  StateEstimation_Bus : Inport  Port=3
  Bus Selector : BusSelector  OutputSignals=omega_OB_B,airdata
  Deflections : Scope  Commented=on  NumInputPorts=3
  Deflections1 : Scope  Commented=on  NumInputPorts=3
  Demux : Demux  Commented=on  Outputs=3
  Demux1 : Demux  Commented=on  Outputs=3
  Demux2 : Demux  Outputs=3
  Demux3 : Demux  Commented=on  Outputs=3
  Gain : Gain  Gain=[1;0;0]
  Mux : Mux  Commented=on  Inputs=2
  Mux1 : Mux  Commented=on  Inputs=2
  Mux2 : Mux  Commented=on  Inputs=2
  Subsystem Reference_SS_4 : Subsystem
  aerodynamic forces FSI : Subsystem
  F_a_B : Outport
  F_p_B : Outport  Port=2
  M_a_B : Outport  Port=3
  tag scope: Aero_forces=global
  wires:
  Bus Selector/2 -> Demux2/1  "<airdata>"
  StateEstimation_Bus/1 -> Bus Selector/1
  throttle/brake/1 -> Gain/1
  Gain/1 -> F_p_B/1
  u_cmd/1 -> Subsystem Reference_SS_4/1(u_cmd), Demux/1
  Bus Selector/1 -> aerodynamic forces FSI/1(omega_b_dist)  "<omega_OB_B>"
  Subsystem Reference_SS_4/1(Act_out_est) -> aerodynamic forces FSI/5(Deflection_act), Demux1/1
  Demux2/1 -> aerodynamic forces FSI/2(vel_air)  "Va"
  Demux2/2 -> aerodynamic forces FSI/3(AoA)  "alpha_in_rad"
  Demux2/3 -> aerodynamic forces FSI/4(Beta_yaw)  "beta_in_rad"
  Demux/1 -> Mux2/1
  Demux/3 -> Mux1/1
  Demux1/1 -> Mux2/2
  Demux/2 -> Mux/1
  Mux/1 -> Deflections/2  "Elevator"
  Mux2/1 -> Deflections/1  "Aileron"
  Mux1/1 -> Deflections/3  "Rudder"
  Demux1/2 -> Mux/2
  Demux1/3 -> Mux1/2
  aerodynamic forces FSI/1(F_a_B) -> [Aero_forces], F_a_B/1
  aerodynamic forces FSI/2(M_a_B) -> Demux3/1, M_a_B/1
  Demux3/1 -> Deflections1/1
  Demux3/2 -> Deflections1/2
  Demux3/3 -> Deflections1/3

== system Dyn_6DoF_v2_0_R2015B/Environment_SS_5/Windshear ==
  DCM : Inport
  altitude : Inport  Port=2
  Math Function : Math  Operator=transpose  SaturateOnIntegerOverflow=on
  Wind Shear Model : Subsystem
  V_shear_mDs : Outport
  wires:
  altitude/1 -> Wind Shear Model/1(Altitude)
  DCM/1 -> Math Function/1
  Math Function/1 -> Wind Shear Model/2(DCM)
  Wind Shear Model/1(Mean Wind) -> V_shear_mDs/1

== system Dyn_6DoF_v2_0_R2015B/Environment_SS_5/wind_field_calc ==
  Altitude : Inport
  Base_windspeed : Inport  Port=2
  1-D Lookup Table : Lookup_n-D  NumberOfTableDimensions=1  BreakpointsForDimension1=ENVMT.wind_height  Table=ENVMT.wind_data  InternalRulePriority=Speed  RndMeth=Simplest  InputSameDT=on
  3ft-->inf : Saturate  Commented=on  UpperLimit=inf  LowerLimit=3
  Length Conversion : Subsystem  Commented=on
  Manual Switch : ManualSwitch  CurrentSetting=0
  Product : Product  Commented=on  Inputs=*/  SaturateOnIntegerOverflow=on  InputSameDT=on  OutDataTypeStr=Inherit: Same as first input
  Product1 : Product  Commented=on  SaturateOnIntegerOverflow=on  InputSameDT=on  OutDataTypeStr=Inherit: Same as first input
  Product2 : Product  SaturateOnIntegerOverflow=on  InputSameDT=on  OutDataTypeStr=Inherit: Same as first input
  Reshape : Reshape  OutputDimensionality=Column vector (2-D)
  Saturation : Saturate  UpperLimit=ENVMT.height_max  LowerLimit=ENVMT.wind_height(1)
  h/z0 : Gain  Commented=on  Gain=1/0.15  SaturateOnIntegerOverflow=on  OutDataTypeStr=Inherit: Same as input  ParamDataTypeStr=Inherit: Same as input
  ln(h/z0) : Math  Commented=on  Operator=log  SaturateOnIntegerOverflow=on
  ln(ref_height/z0) : Math  Commented=on  Operator=log  SaturateOnIntegerOverflow=on
  ref_height/z0 [ft] : Constant  Commented=on  Value=20/0.15  OutDataTypeStr=Inherit: Inherit via back propagation
  Windspeed_altitude : Outport
  wires:
  Altitude/1 -> Saturation/1, Length Conversion/1(in)
  ref_height/z0 [ft]/1 -> ln(ref_height/z0)/1
  h/z0/1 -> ln(h/z0)/1
  Product/1 -> Product1/1
  Manual Switch/1 -> Reshape/1
  Saturation/1 -> 1-D Lookup Table/1  "ijmuiden"
  Base_windspeed/1 -> Product2/2, Product1/2
  Product1/1 -> Manual Switch/1  "log-law"
  Length Conversion/1(out) -> 3ft-->inf/1
  ln(h/z0)/1 -> Product/1
  Reshape/1 -> Windspeed_altitude/1
  1-D Lookup Table/1 -> Product2/1
  ln(ref_height/z0)/1 -> Product/2
  Product2/1 -> Manual Switch/2  "referencce location"
  3ft-->inf/1 -> h/z0/1

== system Dyn_6DoF_v2_0_R2015B/GroundSystem_SS_6/GroundControl ==
  flightMode : Inport
  long : Inport  Port=2
  Chart : Stateflow chart  TreatAsAtomicUnit=on
  Compare To Constant : simulink/Logic and Bit Operations/Compare To Constant  relop===  const=1  OutDataTypeStr=boolean
  Compare To Constant2 : simulink/Logic and Bit Operations/Compare To Constant  relop===  const=6  OutDataTypeStr=boolean
  Compare To Constant3 : simulink/Logic and Bit Operations/Compare To Constant  relop===  const=5  OutDataTypeStr=boolean
  Constant : Constant  Value=0
  Constant1 : Constant  Value=0
  Constant11 : Constant  Value=params.phi0_booth
  Constant9 : Constant  Value=params.transition_phi
  Gain4 : Gain  Gain=pi/180
  Gain7 : Gain  Gain=params.w0_decrease_init_phi0
  Integrator : Integrator  ExternalReset=rising  InitialConditionSource=external
  Logical Operator1 : Logic  Operator=OR  AllPortsSameDT=off  OutDataTypeStr=boolean
  Mux : Mux  Inputs=3
  Select_init_sol_for_pathfollowing : Stateflow chart  TreatAsAtomicUnit=on
  Sum3 : Sum  Inputs=|+-
  Switch : Switch  Criteria=u2 > Threshold
  Switch3 : Switch  Threshold=1
  initial_path_elevation : Constant  Value=params.initial_path_elevation
  path_update : Outport  PortDimensions=[3,1]
  lat_init : Outport  Port=2
  wires:
  Constant1/1 -> Mux/3
  Constant/1 -> Mux/2
  Mux/1 -> path_update/1
  Sum3/1 -> Gain7/1
  Select_init_sol_for_pathfollowing/1(sol_init) -> Gain4/1
  flightMode/1 -> Select_init_sol_for_pathfollowing/2(fm), Compare To Constant3/1, Compare To Constant2/1, Chart/2(fm)
  Compare To Constant2/1 -> Logical Operator1/2
  Switch/1 -> Sum3/1
  Compare To Constant3/1 -> Switch/2
  initial_path_elevation/1 -> Select_init_sol_for_pathfollowing/1(x)
  long/1 -> Chart/1(long)  "long"
  Chart/1(c_out) -> Switch3/2, Compare To Constant/1
  Gain4/1 -> Switch3/3, Integrator/3, lat_init/1, Switch/3
  Integrator/1 -> Sum3/2, Switch3/1
  Compare To Constant/1 -> Logical Operator1/1
  Logical Operator1/1 -> Integrator/2
  Gain7/1 -> Integrator/1
  Switch3/1 -> Mux/1
  Constant9/1 -> Select_init_sol_for_pathfollowing/3(transition_phi)
  Constant11/1 -> Switch/1

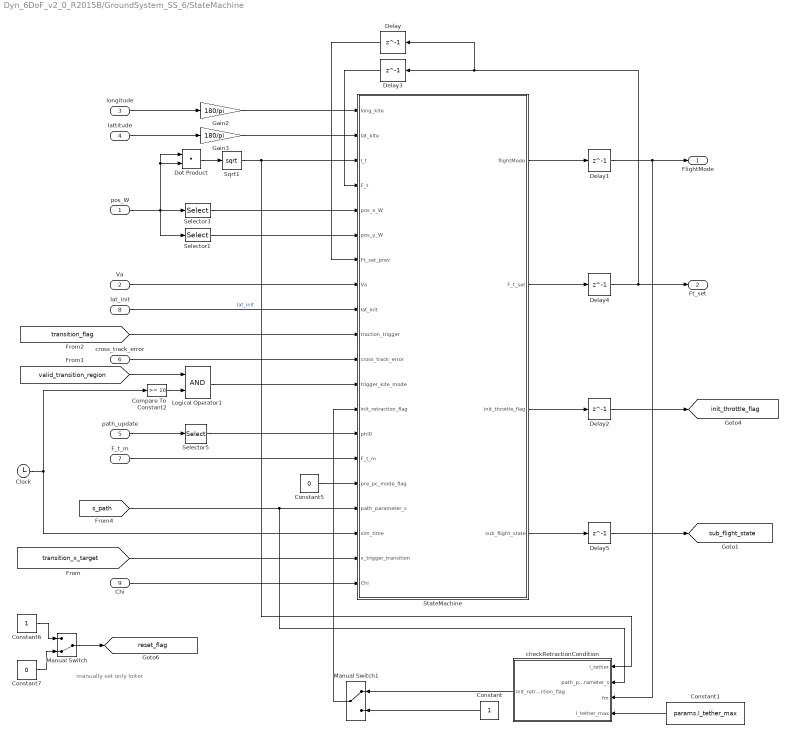
== system Dyn_6DoF_v2_0_R2015B/GroundSystem_SS_6/StateMachine ==
  note: manually set only loiter
  pos_W : Inport
  Va : Inport  Port=2
  longitude : Inport  Port=3
  lattitude : Inport  Port=4
  path_update : Inport  Port=5
  cross_track_error : Inport  Port=6
  F_t_m : Inport  Port=7
  lat_init : Inport  Port=8
  Chi : Inport  Port=9
  Clock : Clock
  Compare To Constant2 : simulink/Logic and Bit Operations/Compare To Constant  relop=>=  const=10  OutDataTypeStr=boolean
  Constant : Constant
  Constant1 : Constant  Value=params.l_tether_max
  Constant5 : Constant  Value=0
  Constant6 : Constant
  Constant7 : Constant  Value=0
  Delay : Delay  DelayLength=1  InitialCondition=100
  Delay1 : Delay  DelayLength=1
  Delay2 : Delay  DelayLength=1  InitialCondition=1
  Delay3 : Delay  DelayLength=1  InitialCondition=100
  Delay4 : Delay  DelayLength=1
  Delay5 : Delay  DelayLength=1  InitialCondition=1
  Dot Product : DotProduct  InputSameDT=on  OutDataTypeStr=Inherit: Inherit via internal rule
  Gain2 : Gain  Gain=180/pi
  Gain3 : Gain  Gain=180/pi
  Logical Operator1 : Logic  AllPortsSameDT=off  OutDataTypeStr=boolean
  Manual Switch : ManualSwitch  CurrentSetting=0
  Manual Switch1 : ManualSwitch
  Selector1 : Selector  InputPortWidth=3  IndexOptions=Index vector (dialog)  Indices=2  OutputSizes=1
  Selector3 : Selector  InputPortWidth=3  IndexOptions=Index vector (dialog)  Indices=1  OutputSizes=1
  Selector5 : Selector  InputPortWidth=3  IndexOptions=Index vector (dialog)  Indices=1  OutputSizes=1
  Sqrt1 : Sqrt  SaturateOnIntegerOverflow=on
  StateMachine : Stateflow chart  TreatAsAtomicUnit=on  mask{F_T_traction_set=params.F_t_traction_set, F_set_retraction=params.F_t_retraction_set*params.F_t_traction_set, l_t_min=params.l_tether_min, l_t_max=params.l_tether_max, a_booth=params.a_booth, b_booth=params.b_booth, lat_trans=0, alpha2=params.ft_smooth_2, crosstrackerror_condition=params.crosstrackerror_condition, Vamin=constr.Va_min, Ft_set_loiter=loiterStates.Ft_set_loiter}
      mask prompts: F_T_traction_set "Traction force"; F_set_retraction "Retraction force"; l_t_min "Min. tether length"; l_t_max "Max. tether length"; a_booth "abooth"; b_booth "bbooth"; alpha2 "interpolation factor retrac 2 trac"
  checkRetractionCondition : Stateflow chart  TreatAsAtomicUnit=on
  FlightMode : Outport
  Ft_set : Outport  Port=2
  tag scope: init_throttle_flag=global, reset_flag=global, sub_flight_state=global
  wires:
  Manual Switch1/1 -> StateMachine/13(init_retraction_flag)
  Constant1/1 -> checkRetractionCondition/4(l_tether_max)
  Va/1 -> StateMachine/8(Va)
  StateMachine/2(F_t_set) -> Delay4/1
  lattitude/1 -> Gain3/1
  longitude/1 -> Gain2/1
  Delay2/1 -> [init_throttle_flag]
  StateMachine/3(init_throttle_flag) -> Delay2/1
  Delay1/1 -> FlightMode/1, checkRetractionCondition/3(fm)
  [valid_transition_region] -> Logical Operator1/1
  Compare To Constant2/1 -> Logical Operator1/2
  Logical Operator1/1 -> StateMachine/12(trigger_kite_mode)
  cross_track_error/1 -> StateMachine/11(cross_track_error)
  Selector1/1 -> StateMachine/6(pos_y_W)
  Delay/1 -> StateMachine/7(Ft_set_prev)
  Dot Product/1 -> Sqrt1/1
  Selector3/1 -> StateMachine/5(pos_x_W)
  pos_W/1 -> Dot Product/1, Dot Product/2, Selector1/1, Selector3/1
  Gain2/1 -> StateMachine/1(long_kite)
  StateMachine/1(flightMode) -> Delay1/1
  Delay3/1 -> StateMachine/4(F_t)
  Selector5/1 -> StateMachine/14(phi0)
  path_update/1 -> Selector5/1
  Gain3/1 -> StateMachine/2(lat_kite)
  Sqrt1/1 -> checkRetractionCondition/1(l_tether), StateMachine/3(l_t)
  Delay4/1 -> Ft_set/1, Delay/1, Delay3/1
  StateMachine/4(sub_flight_state) -> Delay5/1
  F_t_m/1 -> StateMachine/15(F_t_m)
  Constant5/1 -> StateMachine/16(pre_pc_mode_flag)
  [transition_flag] -> StateMachine/10(traction_trigger)
  Constant6/1 -> Manual Switch/1
  Constant7/1 -> Manual Switch/2
  Manual Switch/1 -> [reset_flag]
  Clock/1 -> Compare To Constant2/1, StateMachine/18(sim_time)
  [s_path] -> checkRetractionCondition/2(path_parameter_s), StateMachine/17(path_parameter_s)
  lat_init/1 -> StateMachine/9(lat_init)  "lat_init"
  checkRetractionCondition/1(init_retraction_flag) -> Manual Switch1/1
  Constant/1 -> Manual Switch1/2
  Delay5/1 -> [sub_flight_state]
  [transition_x_target] -> StateMachine/19(x_trigger_transition)
  Chi/1 -> StateMachine/20(Chi)

== system Dyn_6DoF_v2_0_R2015B/ParticleTetherModel/Tether_SS_7 ==
  pos_G_W : Inport
  vel_W : Inport  Port=2
  windVel : Inport  Port=3
  tetherLength : Inport  Port=4
  Delay10 : Delay  DelayLength=1  InitialCondition=zeros(3,1)
  Delay2 : Delay  DelayLength=1  InitialCondition=T.Tn_vect
  Delay3 : Delay  DelayLength=1
  Delay4 : Delay  DelayLength=1  InitialCondition=T.pos_p_init
  Gain1 : Gain  Gain=-1
  Tether_Dynamics : MATLAB Function  TreatAsAtomicUnit=on
  x tether W : Outport
  Ft_Ground : Outport  Port=2
  Ft_Kite : Outport  Port=3
  Error_3D : Outport  Port=4
  wires:
  tetherLength/1 -> Tether_Dynamics/4(tetherLength)
  Delay10/1 -> Ft_Kite/1
  Gain1/1 -> Delay10/1
  Delay3/1 -> Ft_Ground/1
  Delay4/1 -> x tether W/1
  Delay2/1 -> Tether_Dynamics/5("x ")
  Tether_Dynamics/5(x) -> Delay2/1
  windVel/1 -> Tether_Dynamics/3(windVel)
  pos_G_W/1 -> Tether_Dynamics/1(kitePos)
  Tether_Dynamics/1(tetherPos) -> Delay4/1  "x tether W"
  Tether_Dynamics/3(Ft_Kite) -> Gain1/1
  Tether_Dynamics/2(Ft_Ground) -> Delay3/1
  vel_W/1 -> Tether_Dynamics/2(kiteVel)
  Tether_Dynamics/4(Fvec) -> Error_3D/1

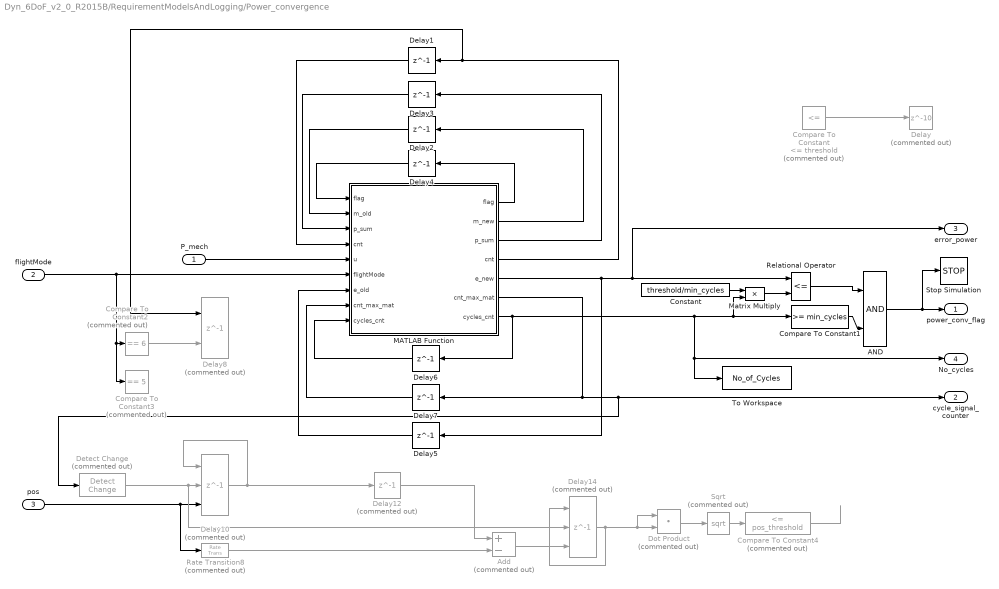
== system Dyn_6DoF_v2_0_R2015B/RequirementModelsAndLogging/Power_convergence ==
  P_mech : Inport
  flightMode : Inport  Port=2
  pos : Inport  Port=3
  AND : Logic  AllPortsSameDT=off  OutDataTypeStr=boolean
  Add : Sum  Commented=on  Inputs=+-
  Compare To Constant : simulink/Logic and Bit Operations/Compare To Constant  Commented=on  relop=<=  const=threshold  OutDataTypeStr=boolean
  Compare To Constant1 : simulink/Logic and Bit Operations/Compare To Constant  relop=>=  const=min_cycles  OutDataTypeStr=boolean
  Compare To Constant2 : simulink/Logic and Bit Operations/Compare To Constant  Commented=on  relop===  const=6  OutDataTypeStr=boolean
  Compare To Constant3 : simulink/Logic and Bit Operations/Compare To Constant  Commented=on  relop===  const=5  OutDataTypeStr=boolean
  Compare To Constant4 : simulink/Logic and Bit Operations/Compare To Constant  Commented=on  relop=<=  const=pos_threshold  OutDataTypeStr=boolean
  Constant : Constant  Value=threshold/min_cycles
  Delay : Delay  Commented=on  DelayLength=10
  Delay{1..4,6..7} (6 alike) : Delay  DelayLength=1  InitialCondition=0
  Delay10 : Delay  Commented=on  DelayLength=1  InitialConditionSource=Input port  InitialCondition=0  ExternalReset=Rising
      settings: InputPortMap=u0,r5,p4
  Delay12 : Delay  Commented=on  DelayLength=1  InitialCondition=0
  Delay14 : Delay  Commented=on  DelayLength=1  InitialConditionSource=Input port  InitialCondition=0  ExternalReset=Rising
      settings: InputPortMap=u0,r5,p4
  Delay5 : Delay  DelayLength=1  InitialCondition=threshold+1000
  Delay8 : Delay  Commented=on  DelayLength=1  InitialCondition=0  ExternalReset=Rising
      settings: InputPortMap=u0,r5
  Detect Change : simulink/Logic and Bit Operations/Detect Change  Commented=on  vinit=0  OutDataTypeStr=boolean
  Dot Product : DotProduct  Commented=on  InputSameDT=on  OutDataTypeStr=Inherit: Inherit via internal rule
  MATLAB Function : MATLAB Function  TreatAsAtomicUnit=on
  Matrix Multiply : Product
  Rate Transition8 : RateTransition  Commented=on  X0=[0;0;0]  OutPortSampleTime=sample_time
  Relational Operator : RelationalOperator  Operator=<=  OutDataTypeStr=boolean
  Sqrt : Sqrt  Commented=on  SaturateOnIntegerOverflow=on
  Stop Simulation : Stop
  To Workspace : ToWorkspace  VariableName=No_of_Cycles  SaveFormat=Timeseries  SampleTime=-1
      settings: MaxDataPoints=1
  power_conv_flag : Outport
  cycle_signal_counter : Outport  Port=2
  error_power : Outport  Port=3
  No_cycles : Outport  Port=4
  wires:
  Delay1/1 -> MATLAB Function/4("cnt ")
  P_mech/1 -> MATLAB Function/5(u)
  MATLAB Function/4(cnt) -> Delay8/1, Delay1/1
  Delay2/1 -> MATLAB Function/2(m_old)
  MATLAB Function/1(flag) -> Delay4/1
  Delay4/1 -> MATLAB Function/1("flag ")
  Delay3/1 -> MATLAB Function/3("p_sum ")
  MATLAB Function/3(p_sum) -> Delay3/1
  MATLAB Function/5(e_new) -> Relational Operator/1, error_power/1, Delay5/1
  Delay5/1 -> MATLAB Function/7(e_old)
  AND/1 -> Stop Simulation/1, power_conv_flag/1
  Delay7/1 -> MATLAB Function/8("cnt_max_mat ")
  MATLAB Function/2(m_new) -> Delay2/1
  MATLAB Function/7(cycles_cnt) -> Compare To Constant1/1, Matrix Multiply/2, No_cycles/1, To Workspace/1, Delay6/1
  Delay6/1 -> MATLAB Function/9("cycles_cnt ")
  Relational Operator/1 -> AND/1
  Compare To Constant1/1 -> AND/2
  Compare To Constant2/1 -> Delay8/2
  Compare To Constant/1 -> Delay/1
  Constant/1 -> Matrix Multiply/1
  Matrix Multiply/1 -> Relational Operator/2
  pos/1 -> Rate Transition8/1, Delay10/3
  Sqrt/1 -> Compare To Constant4/1
  Dot Product/1 -> Sqrt/1
  Delay14/1 -> Delay14/1, Dot Product/1, Dot Product/2
  Rate Transition8/1 -> Add/2
  MATLAB Function/6(cnt_max_mat) -> Detect Change/1, cycle_signal_counter/1, Delay7/1
  Delay10/1 -> Delay12/1, Delay10/1
  flightMode/1 -> MATLAB Function/6(flightMode), Compare To Constant3/1, Compare To Constant2/1
  Add/1 -> Delay14/3
  Detect Change/1 -> Delay14/2, Delay10/2
  Compare To Constant4/1 -> ?
  Delay12/1 -> Add/1

== system Dyn_6DoF_v2_0_R2015B/RequirementModelsAndLogging/Subsystem ==
  In1 : Inport
  Dot Product3 : DotProduct  InputSameDT=on  OutDataTypeStr=Inherit: Inherit via internal rule
  Sqrt1 : Sqrt  SaturateOnIntegerOverflow=on
  Out1 : Outport
  wires:
  In1/1 -> Dot Product3/1, Dot Product3/2
  Sqrt1/1 -> Out1/1
  Dot Product3/1 -> Sqrt1/1

== system Dyn_6DoF_v2_0_R2015B/RequirementModelsAndLogging/Subsystem2 ==
  P_mech : Inport
  Constant7 : Constant
  Delay1 : Delay  DelayLength=1  SampleTime=0.1
  Delay3 : Delay  DelayLength=1  SampleTime=0.1
  Delay4 : Delay  DelayLength=1  InitialCondition=1  SampleTime=0.1
  Divide : Product  Inputs=*/
  Divide1 : Product  Inputs=*/
  Product : Product
  Rate Transition1 : RateTransition  OutPortSampleTime=0.1
  Rate Transition6 : RateTransition  OutPortSampleTime=0.1
  Sum : Sum  Inputs=|+-
  Sum1 : Sum  Inputs=|++
  Sum3 : Sum  Inputs=|++
  Sum4 : Sum  Inputs=|++
  To Workspace : ToWorkspace  Commented=on  VariableName=P_mech  SampleTime=log_sample_time
  mean_Pmech : Outport
  var_Pmech : Outport  Port=2
  wires:
  P_mech/1 -> Rate Transition6/1
  Delay4/1 -> Sum4/2
  Constant7/1 -> Rate Transition1/1
  Divide/1 -> mean_Pmech/1, Sum/2
  Rate Transition1/1 -> Sum4/1
  Sum3/1 -> Divide/1, Delay3/1
  Sum4/1 -> Divide1/2, Delay4/1, Divide/2
  Delay3/1 -> Sum3/2
  Sum/1 -> Product/2, Product/1
  Product/1 -> Sum1/1
  Delay1/1 -> Sum1/2
  Sum1/1 -> Divide1/1, Delay1/1
  Divide1/1 -> var_Pmech/1
  Rate Transition6/1 -> To Workspace/1, Sum/1, Sum3/1  "vel_w_W"

== system Dyn_6DoF_v2_0_R2015B/Subsystem WinchControl_SS_8/PureTorqueControl ==
  F_t_m_grnd : Inport
  retraction_flag : Inport  Port=2
  F_t_set : Inport  Port=3
  theta_dot : Inport  Port=4
  Constant : Constant  Value=0
  Constant4 : Constant  Value=constr.winchParameter.a_max/winchParameter.radius
  Constant5 : Constant  Value=constr.winchParameter.a_min/winchParameter.radius
  Dot Product1 : DotProduct  InputSameDT=on  OutDataTypeStr=Inherit: Inherit via internal rule
  FT set : Scope  NumInputPorts=2
  Gain : Gain  Gain=winchParameter.inertia
  Gain1 : Gain  Gain=winchParameter.inertia
  Gain2 : Gain  Gain=winchParameter.friction
  Gain4 : Gain  Gain=winchParameter.radius
  PI-ForceController : Subsystem
  Saturation Dynamic : simulink/Discontinuities/Saturation Dynamic  OutMin=[]  OutMax=[]  OutDataTypeStr=Inherit: Same as second input  OutDataType=fixdt(1, 16)  OutScaling=2^-10  DoSatur=off
  Sqrt1 : Sqrt  SaturateOnIntegerOverflow=on
  Sum2 : Sum  Inputs=-++
  Sum3 : Sum
  Sum4 : Sum  Inputs=-++
  Sum6 : Sum  Inputs=|-+
  Sum7 : Sum  Inputs=|+-
  torque_cmd : Outport
  wires:
  Sqrt1/1 -> FT set/1, Sum6/2
  retraction_flag/1 -> PI-ForceController/1(RetractionFlag)
  Constant/1 -> Sum3/1
  F_t_set/1 -> FT set/2, Sum6/1
  Gain4/1 -> Sum2/1, Sum4/1
  Constant4/1 -> Gain/1
  Gain/1 -> Sum2/2
  Sum2/1 -> Saturation Dynamic/1
  Constant5/1 -> Gain1/1
  Gain1/1 -> Sum4/2
  Sum4/1 -> Saturation Dynamic/3
  Sum3/1 -> Saturation Dynamic/2, Sum7/2
  Gain2/1 -> Sum4/3, Sum2/3
  Dot Product1/1 -> Sqrt1/1
  F_t_m_grnd/1 -> Dot Product1/1, Dot Product1/2, Gain4/1
  theta_dot/1 -> Gain2/1
  Sum7/1 -> PI-ForceController/2(controlDeficitDue2Sat)
  Sum6/1 -> PI-ForceController/3(e_Ft)
  PI-ForceController/1(TorqueCmd) -> Sum3/2
  Saturation Dynamic/1 -> torque_cmd/1, Sum7/1

== system Dyn_6DoF_v2_0_R2015B/Subsystem WinchControl_SS_8/WinchDynamics ==
  for_tether_tot : Inport
  control_moments : Inport  Port=2
  Discrete-Time Integrator : DiscreteIntegrator  InitialCondition=winchParameter.lj_dot_init  InitialConditionSetting=State (most efficient)  SampleTime=-1  LimitOutput=on  UpperSaturationLimit=constr.winchParameter.v_max/winchParameter.radius  LowerSaturationLimit=constr.winchParameter.v_min/winchParameter.radius  ICPrevOutput=DiscIntNeverNeededParam  ICPrevScaledInput=DiscIntNeverNeededParam
  FrictionCoefficient : Gain  Gain=winchParameter.friction
  Gain{,2..6} (6 alike) : Gain  Gain=winchParameter.radius
  Gain1 : Gain  Gain=1/winchParameter.inertia
  Integrator : Integrator  InitialCondition=winchParameter.winch_angle_init
  Saturation1 : Saturate  UpperLimit=constr.winchParameter.a_max/winchParameter.radius  LowerLimit=constr.winchParameter.a_min/winchParameter.radius
  Sum : Sum  Inputs=+-+
  winch acc : Scope  NumInputPorts=2
  tether_length : Outport
  theta_dot : Outport  Port=2
  winch_acc : Outport  Port=3
  winch_vel : Outport  Port=4
  wires:
  Gain/1 -> tether_length/1
  Gain2/1 -> Sum/1
  Sum/1 -> Gain1/1
  Integrator/1 -> Gain/1  "winch_angle"
  Discrete-Time Integrator/1 -> Gain4/1, FrictionCoefficient/1, theta_dot/1, Integrator/1  "winch_angVel"
  control_moments/1 -> Sum/3
  FrictionCoefficient/1 -> Sum/2
  for_tether_tot/1 -> Gain2/1
  Gain1/1 -> Saturation1/1, Gain5/1, Gain3/1
  Saturation1/1 -> Discrete-Time Integrator/1, Gain6/1  "omega_dot"
  Gain4/1 -> winch_vel/1
  Gain3/1 -> winch_acc/1
  Gain5/1 -> winch acc/1
  Gain6/1 -> winch acc/2
